simulink model "Plant_Characterization"  (R2025a)
settings: Solver=VariableStepAuto  StartTime=0.0  StopTime=t1  RelTol=1e-3
libraries: cstblocks x1
settings Model: Creator=ommor  LastModifiedBy=ommor

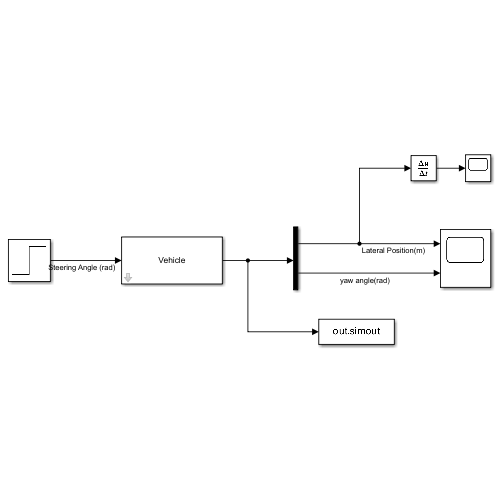
[thumbnail: Simulink's stored preview of the top-level diagram]
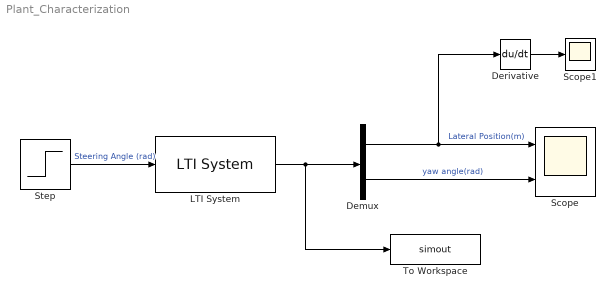
== system Plant_Characterization ==
  Demux : Demux  Outputs=2
  Derivative : Derivative
  LTI System : cstblocks/LTI System  sys=Vehicle  IC=0  PadeOrder=0
  Scope : Scope  NumInputPorts=2
      settings: ActiveDisplayYMinimum=-75.185746533714507  ActiveDisplayYMaximum=676.67171880343074
  Scope1 : Scope
      settings: ActiveDisplayYMinimum=-385.21916091223306  ActiveDisplayYMaximum=2207.9112199573729
  Step : Step  After=pi/6  SampleTime=0
  To Workspace : ToWorkspace  VariableName=simout  SaveFormat=Timeseries  SampleTime=-1
  wires:
  Step/1 -> LTI System/1  "Steering Angle (rad)"
  LTI System/1 -> To Workspace/1, Demux/1
  Demux/1 -> Derivative/1, Scope/1  "Lateral Position(m)"
  Demux/2 -> Scope/2  "yaw angle(rad)"
  Derivative/1 -> Scope1/1
